simulink model "pt8612pll"  (Simulink 5.0)
settings: Solver=ode45  StartTime=0.0  StopTime=4  RelTol=1e-3
values from neighbouring files (symbols this model uses):
  C = 680e-9    (= 6.8e-07)    [PT8612PLLinit.m]    (also in PT8612PLLinit_2.m; PT8612PLLinit_3.m; PT8612PLLinit_4.m; colorimetry_rom.m = [[CrCgCb(1) 0 0];[0 CrCgCb(2) 0];[0 0 CrCgCb(3)]])
  Gi = 1/32    (= 0.03125)    [PT8612PLLinit.m]    (also in PT8612PLLinit_2.m = 0.05)
  Gp = 1/4    (= 0.25)    [PT8612PLLinit.m]    (also in PT8612PLLinit_2.m = 0.025; PT8612PLLinit_4.m = 256)
  R = 100e3    (= 100000)    [PT8612PLLinit.m]    (also in PT8612PLLinit_2.m = 220000; PT8612PLLinit_3.m = 82000; PT8612PLLinit_4.m = 200000; combi_signal.m = [R;ones(red_heigth,spl)])
  Ts = 1/(27e6/91)    (= 3.37037037037e-06)    [PT8612PLLinit.m]
undefined symbols (not defined in the file or in its folder): f0
libraries: simulink x3
settings Model: LastModifiedBy=thh

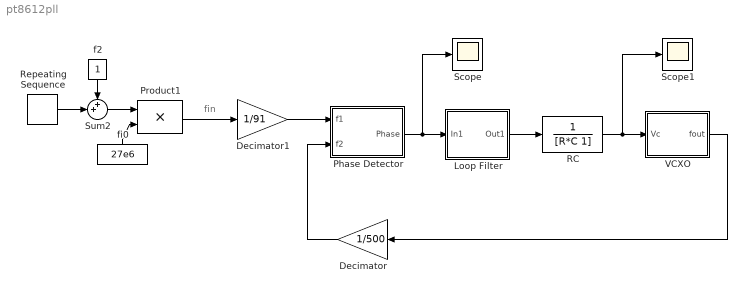
== system pt8612pll ==
  note: fin
  Decimator : Gain  Orientation=left  Gain=1/500  SaturateOnIntegerOverflow=on
  Decimator1 : Gain  Gain=1/91  SaturateOnIntegerOverflow=on
  Loop Filter : Subsystem
  Phase Detector : Subsystem
  Product1 : Product  SaturateOnIntegerOverflow=on
  RC : TransferFcn  Denominator=[R*C 1]
  Repeating Sequence : simulink/Sources/Repeating Sequence  rep_seq_t=[0 0.1 0.1 10]  rep_seq_y=[0 0 1 1]*20e-6
  Scope : Scope
      settings: YMin=5.55112e-017  YMax=1.9
  Scope1 : Scope
      settings: YMin=0.99  YMax=1.05
  Sum2 : Sum  Inputs=++|  SaturateOnIntegerOverflow=on
  VCXO : Subsystem
  f2 : Constant  Orientation=down
  fi0 : Constant  Orientation=up  Value=27e6
  wires:
  Phase Detector/1(Phase) -> Scope/1, Loop Filter/1(In1)
  VCXO/1(fout) -> Decimator/1
  Product1/1 -> Decimator1/1
  fi0/1 -> Product1/2
  f2/1 -> Sum2/1
  Sum2/1 -> Product1/1
  Repeating Sequence/1 -> Sum2/2
  Decimator/1 -> Phase Detector/2(f2)
  Decimator1/1 -> Phase Detector/1(f1)
  Loop Filter/1(Out1) -> RC/1
  RC/1 -> VCXO/1(Vc), Scope1/1

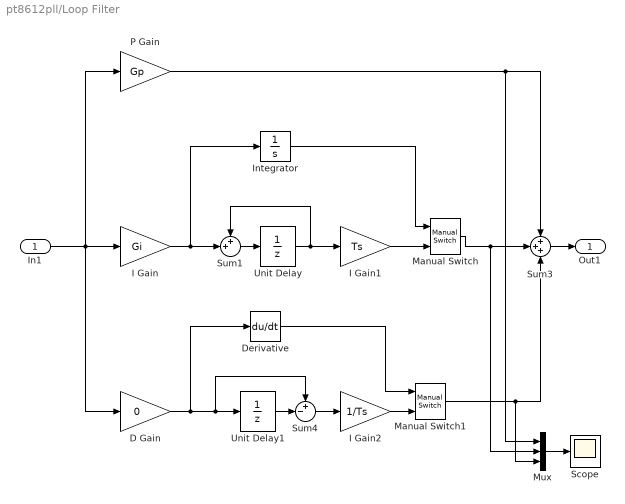
== system pt8612pll/Loop Filter ==
  In1 : Inport
  D Gain : Gain  Gain=0  SaturateOnIntegerOverflow=on
  Derivative : Derivative
  I Gain : Gain  Gain=Gi  SaturateOnIntegerOverflow=on
  I Gain1 : Gain  Gain=Ts  SaturateOnIntegerOverflow=on
  I Gain2 : Gain  Gain=1/Ts  SaturateOnIntegerOverflow=on
  Integrator : Integrator
  Manual Switch : simulink/Signal Routing/Manual Switch  sw=1  action=0
  Manual Switch1 : simulink/Signal Routing/Manual Switch  sw=1  action=0
  Mux : Mux  Inputs=3
  P Gain : Gain  Gain=Gp  SaturateOnIntegerOverflow=on
  Scope : Scope
      settings: YMin=0  YMax=1.1  SaveName=ScopeData2
  Sum1 : Sum  Inputs=++|  SaturateOnIntegerOverflow=on
  Sum3 : Sum  Inputs=+++  SaturateOnIntegerOverflow=on
  Sum4 : Sum  Inputs=+-|  SaturateOnIntegerOverflow=on
  Unit Delay : UnitDelay  SampleTime=-1
  Unit Delay1 : UnitDelay  SampleTime=-1
  Out1 : Outport
  wires:
  Unit Delay/1 -> Sum1/1, I Gain1/1
  Sum1/1 -> Unit Delay/1
  I Gain/1 -> Sum1/2, Integrator/1
  P Gain/1 -> Sum3/1, Mux/1
  In1/1 -> I Gain/1, P Gain/1, D Gain/1
  Sum3/1 -> Out1/1
  Unit Delay1/1 -> Sum4/2
  D Gain/1 -> Unit Delay1/1, Sum4/1, Derivative/1
  Sum4/1 -> I Gain2/1
  Mux/1 -> Scope/1
  I Gain1/1 -> Manual Switch/2
  Manual Switch/1 -> Sum3/2, Mux/2
  Integrator/1 -> Manual Switch/1
  I Gain2/1 -> Manual Switch1/2
  Manual Switch1/1 -> Sum3/3, Mux/3
  Derivative/1 -> Manual Switch1/1

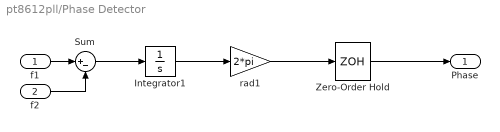
== system pt8612pll/Phase Detector ==
  f1 : Inport
  f2 : Inport  Port=2
  Integrator1 : Integrator
  Sum : Sum  Inputs=|+-  SaturateOnIntegerOverflow=on
  Zero-Order Hold : ZeroOrderHold  SampleTime=Ts
  rad1 : Gain  Gain=2*pi  SaturateOnIntegerOverflow=on
  Phase : Outport
  wires:
  Sum/1 -> Integrator1/1
  Integrator1/1 -> rad1/1
  f1/1 -> Sum/1
  rad1/1 -> Zero-Order Hold/1
  f2/1 -> Sum/2
  Zero-Order Hold/1 -> Phase/1

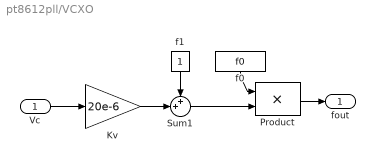
== system pt8612pll/VCXO ==
  Vc : Inport
  Kv : Gain  Gain=20e-6  SaturateOnIntegerOverflow=on
  Product : Product  SaturateOnIntegerOverflow=on
  Sum1 : Sum  Inputs=++|  SaturateOnIntegerOverflow=on
  f0 : Constant  Orientation=down  Value=f0
  f1 : Constant  Orientation=down
  fout : Outport
  wires:
  f0/1 -> Product/1
  f1/1 -> Sum1/1
  Sum1/1 -> Product/2
  Kv/1 -> Sum1/2
  Vc/1 -> Kv/1
  Product/1 -> fout/1
